simulink model "simulink_simulation"  (R2022a)
settings: Solver=ode4  StartTime=0.0  StopTime=4  FixedStep=0.002  RelTol=1e-3
undefined symbols (not defined in the file): K, K_bb, tau
libraries: simulink_extras x1
settings Model: Creator=MLevis  LastModifiedBy=naichenzhao
settings SolverCC: AlgebraicLoopSolver=TrustRegion
settings DataIOCC: InitialState=x0  LoadInitialState=on  ReturnWorkspaceOutputs=off
settings DebuggingCC: UnconnectedInputMsg=warning  UnconnectedOutputMsg=warning  UnconnectedLineMsg=warning  ArithmeticOperatorsInVariantConditions=warning
settings SFSimCC: CustomCodeUndefinedFunction=UseInterfaceOnly
settings CodeAppCC: StateflowObjectComments=on

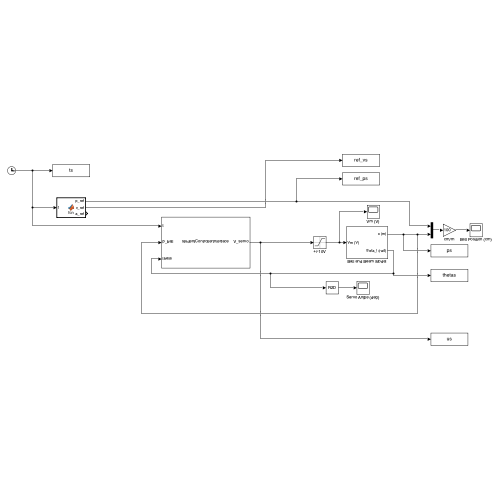
[thumbnail: Simulink's stored preview of the top-level diagram]
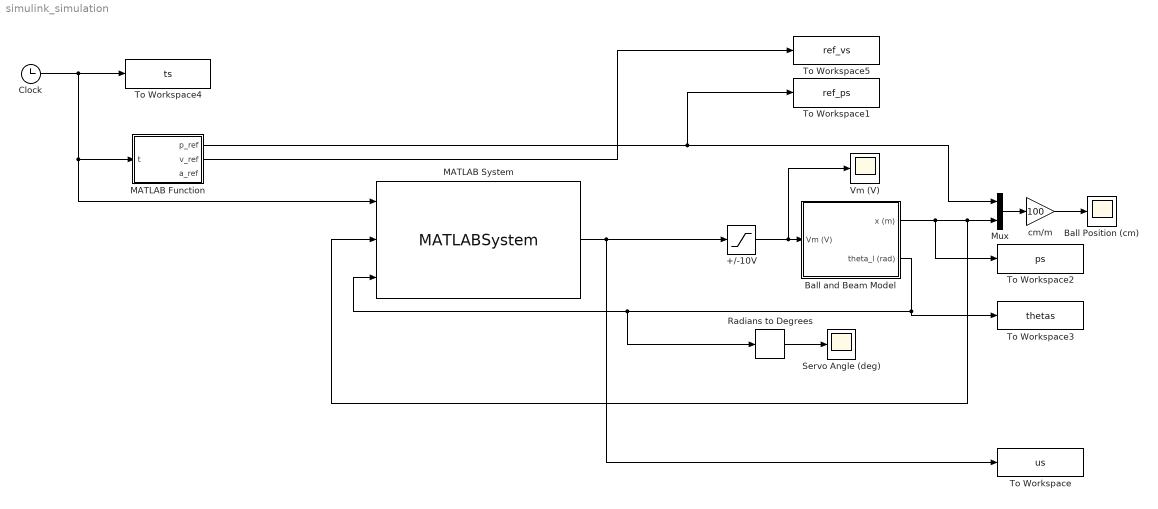
== system simulink_simulation ==
  +/-10V : Saturate  UpperLimit=10  LowerLimit=-10
  Ball Position (cm) : Scope
  Ball and Beam Model : Subsystem
  Clock : Clock
  MATLAB Function : MATLAB Function  TreatAsAtomicUnit=on
  MATLAB System : MATLABSystem  System=studentControllerInterface  SimulateUsing=Code generation
      mask Type: studentControllerInterface
      mask Display:
      | disp('studentControllerInterface');
      | port_label('input',1,'t');
      | port_label('input',2,'p_ball');
      | port_label('input',3,'theta');
      | port_label('output',1,'V_servo');
  Mux : Mux  Inputs=2
  Radians to Degrees : simulink_extras/Transformations/Radians to Degrees
  Servo Angle (deg) : Scope
  To Workspace : ToWorkspace  VariableName=us  SampleTime=0.01
      settings: Save2DSignal=2-D array (concatenate along first dimension)
  To Workspace1 : ToWorkspace  VariableName=ref_ps  SampleTime=0.01
      settings: Save2DSignal=2-D array (concatenate along first dimension)
  To Workspace2 : ToWorkspace  VariableName=ps  SampleTime=0.01
      settings: Save2DSignal=2-D array (concatenate along first dimension)
  To Workspace3 : ToWorkspace  VariableName=thetas  SampleTime=0.01
      settings: Save2DSignal=2-D array (concatenate along first dimension)
  To Workspace4 : ToWorkspace  VariableName=ts  SampleTime=0.01
      settings: Save2DSignal=2-D array (concatenate along first dimension)
  To Workspace5 : ToWorkspace  VariableName=ref_vs  SampleTime=0.01
      settings: Save2DSignal=2-D array (concatenate along first dimension)
  Vm (V) : Scope
  cm/m : Gain  Gain=100
  wires:
  Clock/1 -> To Workspace4/1, MATLAB Function/1(t), MATLAB System/1
  Radians to Degrees/1 -> Servo Angle (deg)/1
  Ball and Beam Model/2(theta_l (rad)) -> To Workspace3/1, MATLAB System/3, Radians to Degrees/1
  cm/m/1 -> Ball Position (cm)/1
  Ball and Beam Model/1(x (m)) -> To Workspace2/1, MATLAB System/2, Mux/2
  MATLAB Function/1(p_ref) -> To Workspace1/1, Mux/1
  +/-10V/1 -> Ball and Beam Model/1(Vm (V)), Vm (V)/1
  Mux/1 -> cm/m/1
  MATLAB System/1 -> To Workspace/1, +/-10V/1
  MATLAB Function/2(v_ref) -> To Workspace5/1

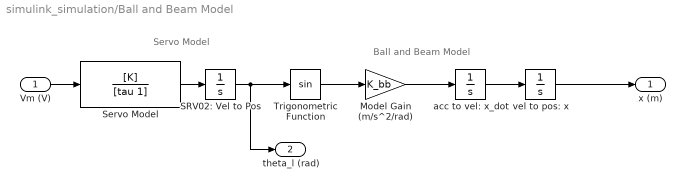
== system simulink_simulation/Ball and Beam Model ==
  note: Servo Model
  note: Ball and Beam Model
  Vm (V) : Inport
  Model Gain (m/s^2/rad) : Gain  Gain=K_bb
  SRV02: Vel to Pos : Integrator
  Servo Model : TransferFcn  Numerator=[K]  Denominator=[tau 1]
  Trigonometric Function : Trigonometry
  acc to vel: x_dot : Integrator
  vel to pos: x : Integrator
  x (m) : Outport
  theta_l (rad) : Outport  Port=2
  wires:
  Servo Model/1 -> SRV02: Vel to Pos/1
  Model Gain (m/s^2/rad)/1 -> acc to vel: x_dot/1
  acc to vel: x_dot/1 -> vel to pos: x/1
  Trigonometric Function/1 -> Model Gain (m/s^2/rad)/1
  Vm (V)/1 -> Servo Model/1
  SRV02: Vel to Pos/1 -> Trigonometric Function/1, theta_l (rad)/1
  vel to pos: x/1 -> x (m)/1

== matlab function simulink_simulation/MATLAB Function ==
  data: t input; p_ref output; v_ref output; a_ref output
function [p_ref, v_ref, a_ref] = fcn(t)

[p_ref, v_ref, a_ref] = get_ref_traj(t);
